simulink model "Open_loop_DC_with_disturbance"  (R2025b)
settings: Solver=VariableStepAuto  StartTime=0.0  StopTime=10.0  RelTol=1e-3
settings Model: Creator=Luqmaan  LastModifiedBy=Luqmaan

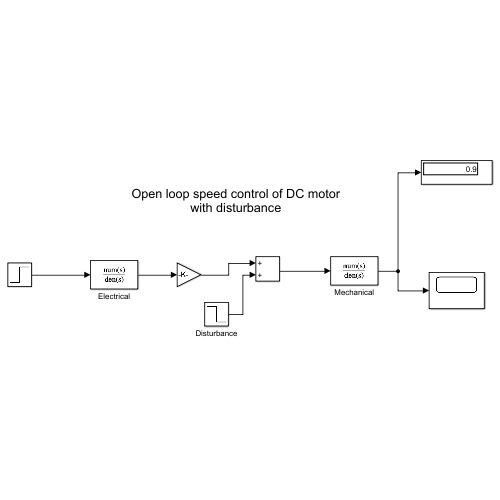
[thumbnail: Simulink's stored preview of the top-level diagram]
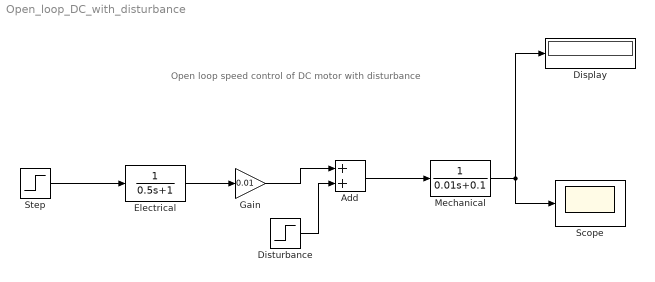
== system Open_loop_DC_with_disturbance ==
  note: Open loop speed control of DC motor with disturbance
  Add : Sum
  Display : Display
  Disturbance : Step  Time=3  After=-0.03  SampleTime=0
  Electrical : TransferFcn  Denominator="[0.5  1]"
  Gain : Gain  Gain=0.01
  Mechanical : TransferFcn  Denominator=[0.01 0.1]
  Scope : Scope
      settings: ActiveDisplayYMinimum=-5.4902982936458571  ActiveDisplayYMaximum=5.3360560148953073
  Step : Step  After=12  SampleTime=0
  wires:
  Mechanical/1 -> Display/1, Scope/1
  Gain/1 -> Add/1
  Step/1 -> Electrical/1
  Electrical/1 -> Gain/1
  Add/1 -> Mechanical/1
  Disturbance/1 -> Add/2
